simulink library "atmoDrag_lib"  (R2018b)
settings: Solver=VariableStepAuto  StartTime=0.0  StopTime=10.0  RelTol=1e-3
libraries: aerolibatmos2 x1, time_Lib x1
settings Model: Creator=Kate  LastModifiedBy=devantormey

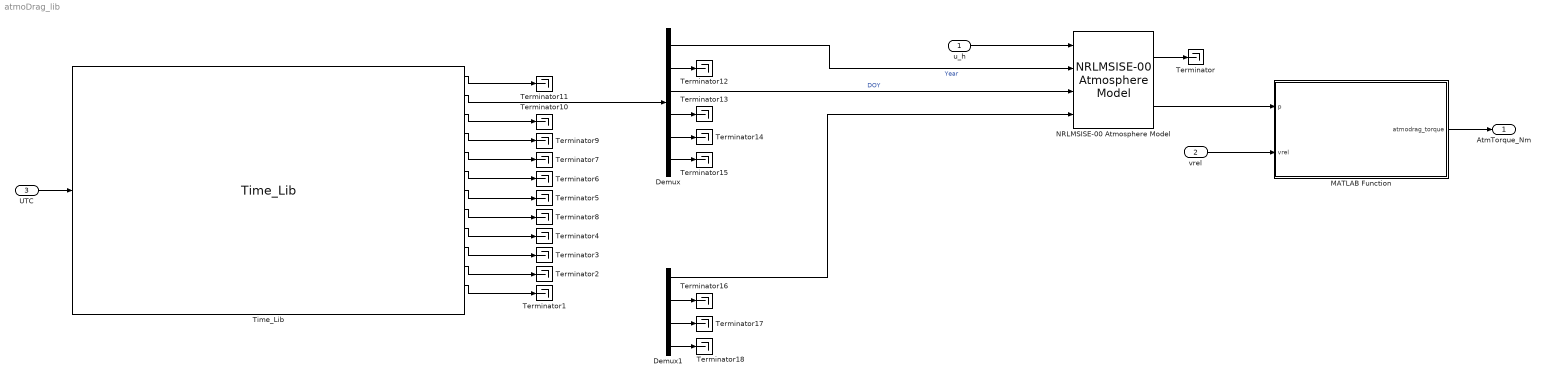
== system atmoDrag_lib ==
  u_h : Inport
  "vrel " : Inport  Port=2
  UTC : Inport  Port=3
  Demux : Demux  Outputs=6
  Demux1 : Demux
  MATLAB Function : MATLAB Function  TreatAsAtomicUnit=on
  NRLMSISE-00 Atmosphere Model : aerolibatmos2/NRLMSISE-00 Atmosphere Model  units=Metric (MKS)  lst_input=off  flux_ap_input=off  flags_input=Internal  flags=ones(1,23)  oxygen_in=off  action=Warning
      settings: SourceProductName=Aerospace Blockset  SourceProductBaseCode=AE
  Terminator{,1..18} (19 alike) : Terminator
  "Time_Lib " : time_Lib/Time_Lib    SystemSampleTime=-1
  AtmTorque_Nm : Outport
  wires:
  NRLMSISE-00 Atmosphere Model/2 -> MATLAB Function/1(p)
  "vrel "/1 -> MATLAB Function/2(vrel)
  Demux/2 -> Terminator12/1
  Demux/5 -> Terminator14/1
  Demux/6 -> Terminator15/1
  NRLMSISE-00 Atmosphere Model/1 -> Terminator/1
  Demux/4 -> Terminator13/1
  Demux/1 -> NRLMSISE-00 Atmosphere Model/2  "Year"
  Demux/3 -> NRLMSISE-00 Atmosphere Model/3  "DOY"
  u_h/1 -> NRLMSISE-00 Atmosphere Model/1
  Demux1/1 -> NRLMSISE-00 Atmosphere Model/4
  Demux1/2 -> Terminator16/1
  Demux1/4 -> Terminator18/1
  Demux1/3 -> Terminator17/1
  "Time_Lib "/2 -> Demux/1
  "Time_Lib "/1 -> Terminator11/1
  "Time_Lib "/3 -> Terminator10/1
  "Time_Lib "/4 -> Terminator9/1
  "Time_Lib "/5 -> Terminator7/1
  "Time_Lib "/6 -> Terminator6/1
  "Time_Lib "/7 -> Terminator5/1
  "Time_Lib "/8 -> Terminator8/1
  "Time_Lib "/9 -> Terminator4/1
  "Time_Lib "/10 -> Terminator3/1
  "Time_Lib "/11 -> Terminator2/1
  "Time_Lib "/12 -> Terminator1/1
  UTC/1 -> "Time_Lib "/1
  MATLAB Function/1(atmodrag_torque) -> AtmTorque_Nm/1

== matlab function atmoDrag_lib/MATLAB Function ==
  data: p input; atmodrag_torque output; vrel input
function atmodrag_torque = atmoDrag(p,vrel)
%Author Kate Williams
%Date created 2/21/2019
%function consists of basic atospheric equation

%drag in units of newtons, a 3D vector
%den=density, gathered from density model kg/m^3
%Cd = coeficent of drag, dimensionless
%A=exposed cross sectional area, m^2
%m=mass of cubsat, kg
%vrel= relative velocity m/s^2
%unitV= unit vector of relative velocity

%cubesat parameters
A= 0.1*0.3; %m^2 of a 3U cubesat reference area
m=4; %kg, this is max mass allowed, final mass yet to be determined
Cd=2.2;% standard for 3U cubesat
%Cd = (1+2/3*sqrt(1-alpha)*sin(theta))*sin(theta)
%https://apps.dtic.mil/dtic/tr/fulltext/u2/a285118.pdf pg 16
%http://citeseerx.ist.psu.edu/viewdoc/download?doi=10.1.1.588.3019&rep=rep1&type=pdf

vrelMag=sqrt(sum(vrel.*vrel));
unitV=vrel/vrelMag; %direction of the drag

%below drag equation from vallado pg 551 eq8-28
atmodrag_N = -0.5*p*(Cd*A/m)*vrelMag^2*unitV; %drag occurs in opposite direction of velocity

%covert to torque N*m
atmodrag_torque=atmodrag_N*0.15;%force*0.5*maxlength of cubesate = 0.5*30cm
